simulink model "Simulink_Simulation"  (R2024b)
settings: Solver=VariableStepAuto  StartTime=0.0  StopTime=0.3  RelTol=1e-3
libraries: cstblocks x9
settings Model: Creator=janic  LastModifiedBy=janic

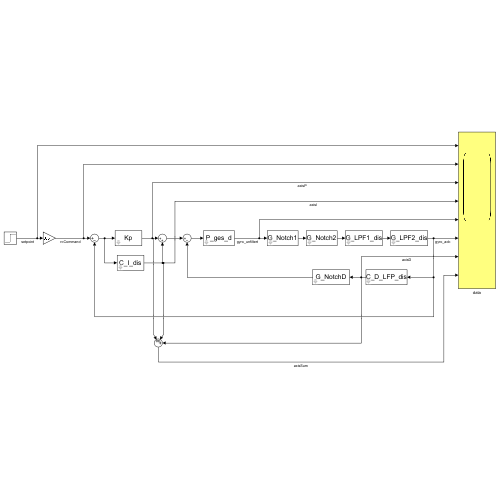
[thumbnail: Simulink's stored preview of the top-level diagram]
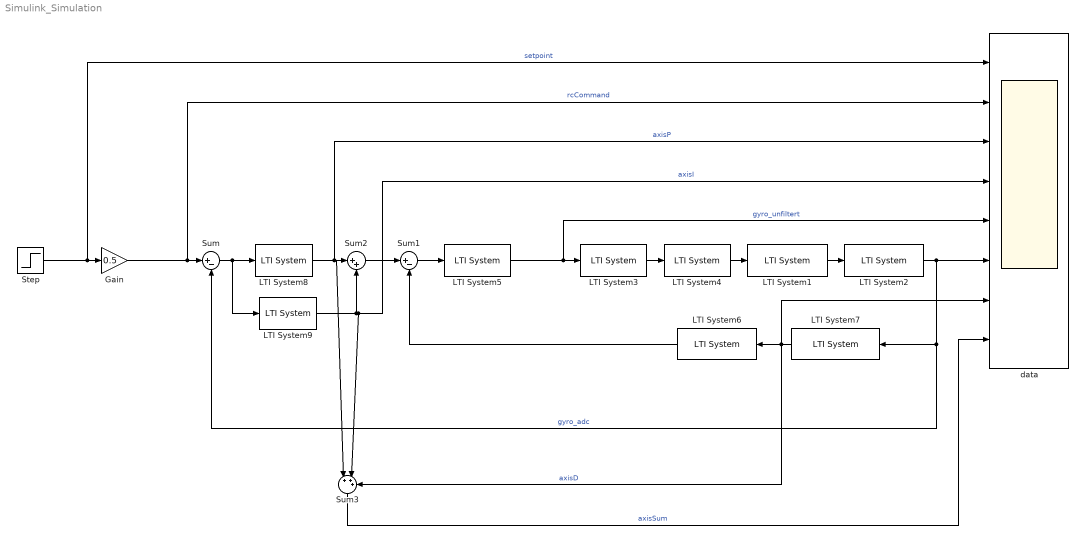
== system Simulink_Simulation ==
  Gain : Gain  Gain=0.5
  LTI System1 : cstblocks/LTI System  sys=G_LPF1_dis  IC=[]  PadeOrder=0
  LTI System2 : cstblocks/LTI System  sys=G_LPF2_dis  IC=[]  PadeOrder=0
  LTI System3 : cstblocks/LTI System  sys=G_Notch1  IC=[]  PadeOrder=0
  LTI System4 : cstblocks/LTI System  sys=G_Notch2  IC=[]  PadeOrder=0
  LTI System5 : cstblocks/LTI System  sys=P_ges_d  IC=[]  PadeOrder=0
  LTI System6 : cstblocks/LTI System  sys=G_NotchD  IC=[]  PadeOrder=0
  LTI System7 : cstblocks/LTI System  sys=C_D_LFP_dis  IC=[]  PadeOrder=0
  LTI System8 : cstblocks/LTI System  sys=Kp  IC=[]  PadeOrder=0
  LTI System9 : cstblocks/LTI System  sys=C_I_dis  IC=[]  PadeOrder=0
  Step : Step  Time=0.05  After=2  SampleTime=0
  Sum : Sum  Inputs=|+-
  Sum1 : Sum  Inputs=|+-
  Sum2 : Sum  Inputs=|++
  Sum3 : Sum  Inputs=|+++
  data : Scope  NumInputPorts=8
      settings: CopyFcn=try ZHAWcbfcn('copyScope'); end  NameChangeFcn=try ZHAWcbfcn('namechangeScope'); end
  wires:
  Step/1 -> data/1, Gain/1  "setpoint"
  Sum/1 -> LTI System9/1, LTI System8/1
  LTI System1/1 -> LTI System2/1
  LTI System3/1 -> LTI System4/1
  Sum1/1 -> LTI System5/1
  LTI System7/1 -> data/7, Sum3/3, LTI System6/1  "axisD"
  LTI System6/1 -> Sum1/2
  LTI System2/1 -> data/6, LTI System7/1, Sum/2  "gyro_adc"
  Sum2/1 -> Sum1/1
  LTI System5/1 -> LTI System3/1, data/5  "gyro_unfiltert"
  LTI System4/1 -> LTI System1/1
  LTI System8/1 -> Sum3/1, data/3, Sum2/1  "axisP"
  LTI System9/1 -> Sum3/2, data/4, Sum2/2  "axisI"
  Gain/1 -> data/2, Sum/1  "rcCommand"
  Sum3/1 -> data/8  "axisSum"
